simulink model "lazocerradoparaK"  (R2021a)
settings: Solver=FixedStepAuto  StartTime=0.0  StopTime=200  FixedStep=1e-3  RelTol=1e-3
settings Model: Creator=Royer  LastModifiedBy=Royer

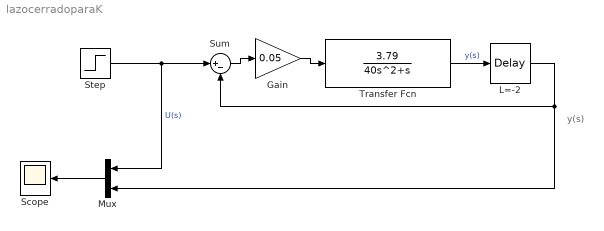
== system lazocerradoparaK ==
  note: y(s)
  Gain : Gain  Gain=0.05
  L=-2 : TransportDelay  DelayTime=2
  Mux : Mux  Inputs=2
  Scope : Scope
  Step : Step  SampleTime=0
  Sum : Sum  Inputs=|+-
  Transfer Fcn : TransferFcn  Numerator=3.79  Denominator=[40 1 0]
  wires:
  Transfer Fcn/1 -> L=-2/1  "y(s)"
  Step/1 -> Sum/1, Mux/1  "U(s)"
  Mux/1 -> Scope/1
  L=-2/1 -> Mux/2, Sum/2
  Sum/1 -> Gain/1
  Gain/1 -> Transfer Fcn/1
